simulink model "AOO"  (R2022a)
settings: Solver=FixedStepAuto  StartTime=0.0  StopTime=1  FixedStep=1e-3  RelTol=1e-3  EnableMultiTasking=on
undefined symbols (not defined in the file or in its folder): D10, D11, D12, D2, D4, D5, D7, D8, D9, PTA0, PTA2, PTB23, PTB9, PTC3, PTC4, PTD0, PTD2, PTD3
libraries: frdmk64flib x9, sldrtlib x1
settings Model: ExtModeTrigDuration=5  Creator=cathe  LastModifiedBy=cathe
settings OptimizationCC: EnhancedBackFolding=on  PassReuseOutputArgsAs=Individual arguments  ZeroExternalMemoryAtStartup=off  ZeroInternalMemoryAtStartup=off  MaxStackSize=64  OptimizeBlockOrder=speed  DifferentSizesBufferReuse=on  OptimizationCustomize=off  EfficientTunableParamExpr=on
settings DebuggingCC: ParameterTunabilityLossMsg=error
settings HardwareCC: ProdBitPerPointer=32  ProdBitPerSizeT=32  ProdBitPerPtrDiffT=32  ProdLargestAtomicInteger=Long  ProdLargestAtomicFloat=Double  ProdWordSize=32  ProdHWDeviceType=ARM Compatible->ARM Cortex
settings SFSimCC: MATLABDynamicMemAlloc=off
settings RTWCC: SystemTargetFile=ert.tlc  HardwareBoard=NXP FRDM-K64F  TLCOptions="-aInlineSetEventsForThisBaseRateFcn=TLC_FALSE -aSuppressMultiTaskScheduler=TLC_FALSE  -aRateBasedStepFcn=0"  TemplateMakefile=ert_default_tmf  Toolchain=GNU Tools for ARM Embedded Processors
settings CodeAppCC: ForceParamTrailComments=on  IgnoreCustomStorageClasses=off  OperatorAnnotations=on  SimulinkDataObjDesc=on  SFDataObjDesc=on  InsertBlockDesc=on
settings ERTTargetCC: ExtModeTransport=4  ExtModeMexFile=sendToCommService

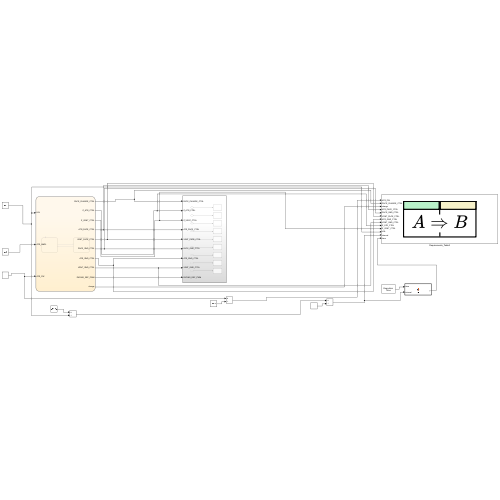
[thumbnail: Simulink's stored preview of the top-level diagram]
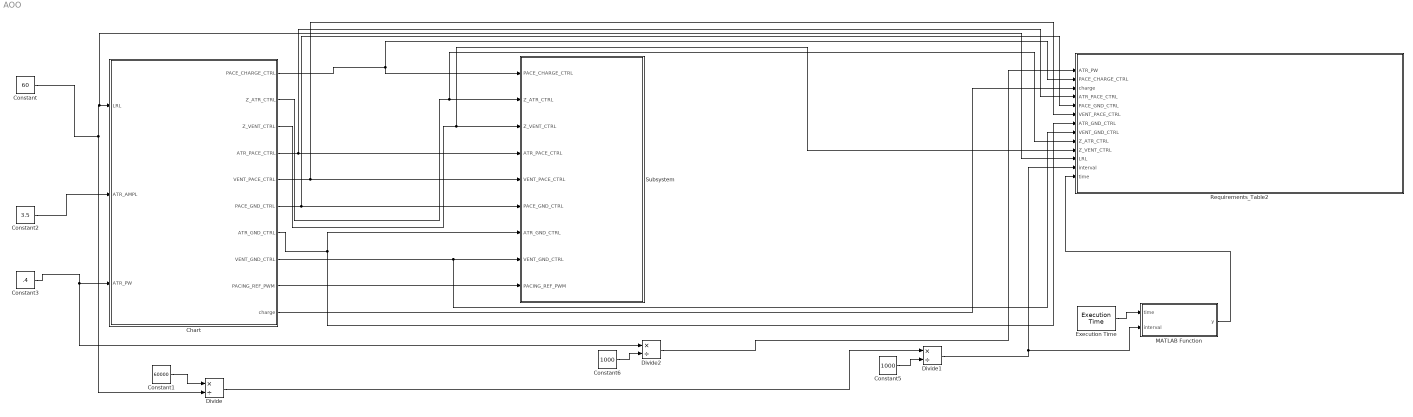
== system AOO ==
  Chart : Stateflow chart  TreatAsAtomicUnit=on
  Constant : Constant  Value=60
  Constant1 : Constant  Value=60000
  Constant2 : Constant  Value=3.5
  Constant3 : Constant  Value=.4
  Constant5 : Constant  Value=1000
  Constant6 : Constant  Value=1000
  Divide : Product  Inputs=*/
  Divide1 : Product  Inputs=*/
  Divide2 : Product  Inputs=*/
  Execution Time : sldrtlib/Target Profiling/Execution Time  ShowTaskTimes=off
      settings: SourceProductBaseCode=WT
  MATLAB Function : MATLAB Function  TreatAsAtomicUnit=on
  Requirements_Table2 : Requirements Table  TreatAsAtomicUnit=on
  Subsystem : Subsystem
  wires:
  Constant2/1 -> Chart/2(ATR_AMPL)
  Constant3/1 -> Divide2/1, Chart/3(ATR_PW)
  Chart/1(PACE_CHARGE_CTRL) -> Requirements_Table2/2(PACE_CHARGE_CTRL), Subsystem/1(PACE_CHARGE_CTRL)
  Chart/2(Z_ATR_CTRL) -> Requirements_Table2/9(Z_ATR_CTRL), Subsystem/2(Z_ATR_CTRL)
  Chart/3(Z_VENT_CTRL) -> Requirements_Table2/10(Z_VENT_CTRL), Subsystem/3(Z_VENT_CTRL)
  Chart/4(ATR_PACE_CTRL) -> Requirements_Table2/4(ATR_PACE_CTRL), Subsystem/4(ATR_PACE_CTRL)
  Chart/5(VENT_PACE_CTRL) -> Requirements_Table2/6(VENT_PACE_CTRL), Subsystem/5(VENT_PACE_CTRL)
  Chart/6(PACE_GND_CTRL) -> Requirements_Table2/5(PACE_GND_CTRL), Subsystem/6(PACE_GND_CTRL)
  Chart/7(ATR_GND_CTRL) -> Requirements_Table2/7(ATR_GND_CTRL), Subsystem/7(ATR_GND_CTRL)
  Chart/8(VENT_GND_CTRL) -> Requirements_Table2/8(VENT_GND_CTRL), Subsystem/8(VENT_GND_CTRL)
  Constant1/1 -> Divide/1
  Constant5/1 -> Divide1/2
  Constant6/1 -> Divide2/2
  Divide2/1 -> Requirements_Table2/1(ATR_PW)
  Chart/9(PACING_REF_PWM) -> Subsystem/9(PACING_REF_PWM)
  Chart/10(charge) -> Requirements_Table2/3(charge)
  Constant/1 -> Requirements_Table2/11(LRL), Chart/1(LRL), Divide/2
  Divide/1 -> Divide1/1
  Divide1/1 -> MATLAB Function/2(interval), Requirements_Table2/12(interval)
  Execution Time/1 -> MATLAB Function/1(time)
  MATLAB Function/1(y) -> Requirements_Table2/13(time)

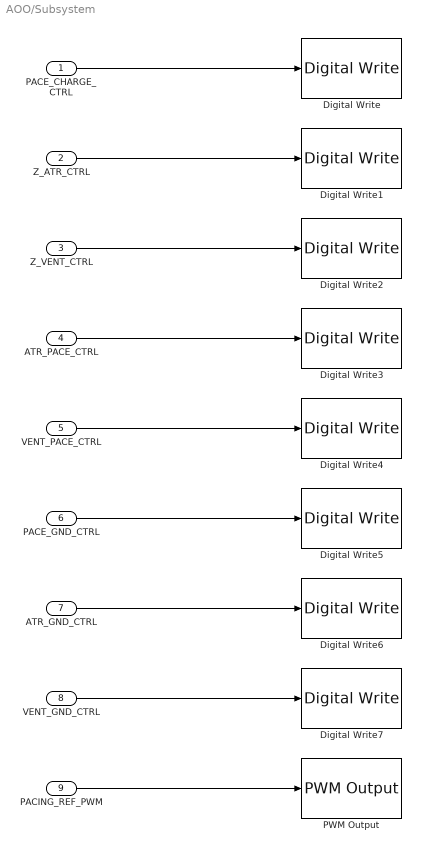
== system AOO/Subsystem ==
  PACE_CHARGE_CTRL : Inport
  Z_ATR_CTRL : Inport  Port=2
  Z_VENT_CTRL : Inport  Port=3
  ATR_PACE_CTRL : Inport  Port=4
  VENT_PACE_CTRL : Inport  Port=5
  PACE_GND_CTRL : Inport  Port=6
  ATR_GND_CTRL : Inport  Port=7
  VENT_GND_CTRL : Inport  Port=8
  PACING_REF_PWM : Inport  Port=9
  Digital Write : frdmk64flib/Digital Write  Whichpin=PTB9 (D2)
  Digital Write1 : frdmk64flib/Digital Write  Whichpin=PTB23 (D4)
  Digital Write2 : frdmk64flib/Digital Write  Whichpin=PTC3 (D7)
  Digital Write3 : frdmk64flib/Digital Write  Whichpin=PTA0 (D8)
  Digital Write4 : frdmk64flib/Digital Write  Whichpin=PTC4 (D9)
  Digital Write5 : frdmk64flib/Digital Write  Whichpin=PTD0 (D10)
  Digital Write6 : frdmk64flib/Digital Write  Whichpin=PTD2 (D11)
  Digital Write7 : frdmk64flib/Digital Write  Whichpin=PTD3 (D12)
  PWM Output : frdmk64flib/PWM Output  Whichpin=PTA2 (D5)  InitialFrequency=2000  InitialDutyCycle=0
  wires:
  PACE_CHARGE_CTRL/1 -> Digital Write/1
  Z_ATR_CTRL/1 -> Digital Write1/1
  Z_VENT_CTRL/1 -> Digital Write2/1
  ATR_PACE_CTRL/1 -> Digital Write3/1
  VENT_PACE_CTRL/1 -> Digital Write4/1
  PACE_GND_CTRL/1 -> Digital Write5/1
  ATR_GND_CTRL/1 -> Digital Write6/1
  VENT_GND_CTRL/1 -> Digital Write7/1
  PACING_REF_PWM/1 -> PWM Output/1

== matlab function AOO/MATLAB Function ==
  data: time input; y output; interval input
function y = fcn(time, interval)

y = time;

while time>interval
    y = y - interval;
end

== stateflow chart AOO/Chart ==
  state CHARGING_DISCHARGING
    entry:
    charge = true;
    et = 0;
    %DISCHARGING C21
    PACE_GND_CTRL = true;
    VENT_PACE_CTRL = false;
    Z_ATR_CTRL = false;
    Z_VENT_CTRL = false;
    ATR_PACE_CTRL = false;
    ATR_GND_CTRL = true;
    VENT_GND_CTRL = false;
    %CHARGING C22
    PACING_REF_PWM = 100*ATR_AMPL/5;
    PACE_CHARGE_CTRL = true;
  state PACE_ATR
    entry:
    charge = false;
    et = 60000/LRL-ATR_PW;
    PACE_CHARGE_CTRL = false;
    PACE_GND_CTRL = true;
    ATR_PACE_CTRL = true;
    ATR_GND_CTRL = false;
    Z_ATR_CTRL = false;
    Z_VENT_CTRL = false;
    VENT_GND_CTRL = false;
    VENT_PACE_CTRL = false;
  (default) -> CHARGING_DISCHARGING
  CHARGING_DISCHARGING -> PACE_ATR : [after(60000/LRL-ATR_PW, msec)]
  PACE_ATR -> CHARGING_DISCHARGING : [after(ATR_PW,msec)]
  data: LRL input; ATR_AMPL input; ATR_PW input; PACE_CHARGE_CTRL output; Z_ATR_CTRL output; Z_VENT_CTRL output; ATR_PACE_CTRL output; VENT_PACE_CTRL output; PACE_GND_CTRL output; ATR_GND_CTRL output; VENT_GND_CTRL output; PACING_REF_PWM output; charge output boolean; et local

== stateflow chart AOO/Requirements_Table2 ==
  (default) -> (junction 1073744464)
  (junction 1073744464) -> (junction 1073744465) : {
      | % SF_REQ_REV_07
      | }
  (junction 1073744465) -> (junction 1073744467) : {
      | % HEADER_ASSIGNMENTS
      |
      | }
  (junction 1073744467) -> (junction 1073744469) : {
      | % START_A_4
      | }
  (junction 1073744469) -> (junction 1073744471) : {
      | }
  (junction 1073744471) -> (junction 1073744473)
  (junction 1073744473) -> (junction 1073744475) : {
      | }
  (junction 1073744475) -> (junction 1073744477) : {
      | % END_A_4
      | }
  (junction 1073744477) -> (junction 1073744479) : {
      | % START_R_16
      | }
  (junction 1073744479) -> (junction 1073744481) : {
      | }
  (junction 1073744481) -> (junction 1073744483)
  (junction 1073744483) -> (junction 1073744485) [order 1] : [(charge == true) && (time < interval - ATR_PW)]
  (junction 1073744483) -> (junction 1073744491) [order 2]
  (junction 1073744485) -> (junction 1073744487) : {
      | reqtable_postcondition((((PACE_GND_CTRL) == (true))) && (((PACE_CHARGE_CTRL) == (true))) && (((VENT_PACE_CTRL) == (false))) && (((ATR_PACE_CTRL) == (false))) && (((VENT_GND_CTRL) == (false))) && (((ATR_GND_CTRL) == (true))) && (((Z_VENT_CTRL) == (false))) && (((Z_ATR_CTRL) == (false))), 'R:1');
      |
      |
      | }
  (junction 1073744487) -> (junction 1073744489) : {
      | }
  (junction 1073744489) -> (junction 1073744491)
  (junction 1073744491) -> (junction 1073744493)
  (junction 1073744493) -> (junction 1073744495) : {
      | % END_R_16
      | }
  (junction 1073744495) -> (junction 1073744497) : {
      | % START_R_19
      | }
  (junction 1073744497) -> (junction 1073744499) : {
      | }
  (junction 1073744499) -> (junction 1073744501)
  (junction 1073744501) -> (junction 1073744503) [order 1] : [( charge == false) && (interval - ATR_PW <= time <= interval)]
  (junction 1073744501) -> (junction 1073744509) [order 2]
  (junction 1073744503) -> (junction 1073744505) : {
      | reqtable_postcondition((((PACE_GND_CTRL) == (true))) && (((PACE_CHARGE_CTRL) == (false))) && (((VENT_PACE_CTRL) == (false))) && (((ATR_PACE_CTRL) == (true))) && (((VENT_GND_CTRL) == (false))) && (((ATR_GND_CTRL) == (false))) && (((Z_VENT_CTRL) == (false))) && (((Z_ATR_CTRL) == (false))), 'R:2');
      |
      |
      | }
  (junction 1073744505) -> (junction 1073744507) : {
      | }
  (junction 1073744507) -> (junction 1073744509)
  (junction 1073744509) -> (junction 1073744511)
  (junction 1073744511) -> (junction 1073744513) : {
      | % END_R_19
      | }
  data: ATR_PW input double; PACE_CHARGE_CTRL input; charge input boolean; ATR_PACE_CTRL input boolean; PACE_GND_CTRL input boolean; VENT_PACE_CTRL input boolean; ATR_GND_CTRL input boolean; VENT_GND_CTRL input boolean; Z_ATR_CTRL input boolean; Z_VENT_CTRL input boolean; LRL input; interval input double; time input
